simulink model "ex1"  (R2022b)
settings: Solver=VariableStepAuto  StartTime=0.0  StopTime=10.0  RelTol=1e-3
settings Model: Creator=ThinkPad  LastModifiedBy=ThinkPad

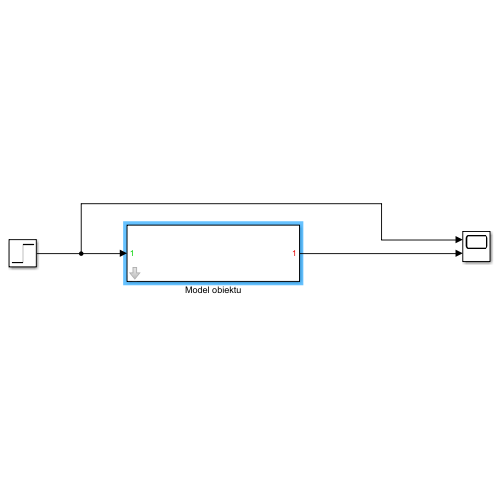
[thumbnail: Simulink's stored preview of the top-level diagram]
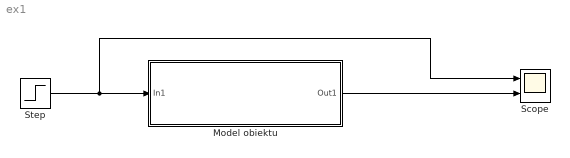
== system ex1 ==
  Model obiektu : Subsystem  mask{wn=1, z=0.5}
      mask prompts: wn "wn = częstotliwość drgań własnych"
  Scope : Scope  NumInputPorts=2
  Step : Step  Time=0  SampleTime=0
  wires:
  Step/1 -> Model obiektu/1(In1), Scope/1
  Model obiektu/1(Out1) -> Scope/2

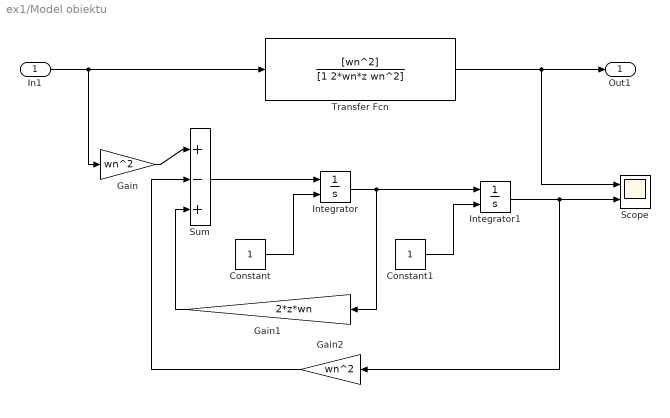
== system ex1/Model obiektu ==
  In1 : Inport
  Constant : Constant
  Constant1 : Constant
  Gain : Gain  Gain=wn^2
  Gain1 : Gain  Gain=2*z*wn
  Gain2 : Gain  Gain=wn^2
  Integrator : Integrator  InitialConditionSource=external
  Integrator1 : Integrator  InitialConditionSource=external
  Scope : Scope  NumInputPorts=2
  Sum : Sum  Inputs=|+-+
  Transfer Fcn : TransferFcn  Numerator=[wn^2]  Denominator=[1 2*wn*z wn^2]
  Out1 : Outport
  wires:
  In1/1 -> Gain/1, Transfer Fcn/1
  Transfer Fcn/1 -> Scope/1, Out1/1
  Gain/1 -> Sum/1
  Sum/1 -> Integrator/1
  Gain1/1 -> Sum/3
  Gain2/1 -> Sum/2
  Constant/1 -> Integrator/2
  Integrator/1 -> Gain1/1, Integrator1/1
  Constant1/1 -> Integrator1/2
  Integrator1/1 -> Gain2/1, Scope/2
